simulink model "n_ordre"  (R2021b)
settings: Solver=VariableStepAuto  StartTime=0.0  StopTime=10.0  RelTol=1e-3
libraries: cstblocks x4
settings Model: Creator=sarmeegan  LastModifiedBy=sarmeegan

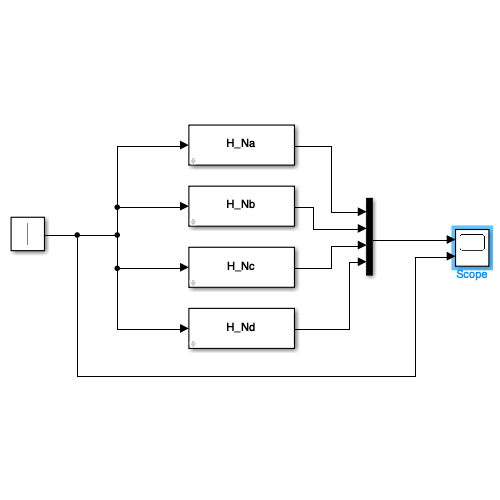
[thumbnail: Simulink's stored preview of the top-level diagram]
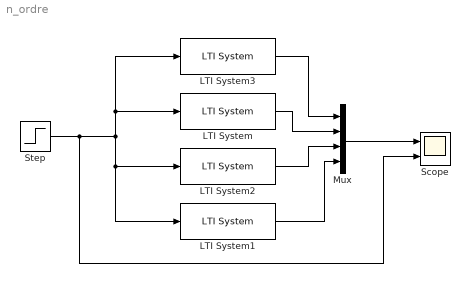
== system n_ordre ==
  LTI System : cstblocks/LTI System  sys=H_Nb  IC=[]
  LTI System1 : cstblocks/LTI System  sys=H_Nd  IC=[]
  LTI System2 : cstblocks/LTI System  sys=H_Nc  IC=[]
  LTI System3 : cstblocks/LTI System  sys=H_Na  IC=[]
  Mux : Mux
  Scope : Scope  NumInputPorts=2
  Step : Step  Time=0  SampleTime=0
  wires:
  Step/1 -> Scope/2, LTI System1/1, LTI System2/1, LTI System/1, LTI System3/1
  LTI System3/1 -> Mux/1
  LTI System/1 -> Mux/2
  LTI System2/1 -> Mux/3
  LTI System1/1 -> Mux/4
  Mux/1 -> Scope/1
